simulink model "simulacaoOrientacaoESC"  (R2015a)
settings: Solver=ode4  StartTime=0.0  StopTime=60  FixedStep=0.0001  RelTol=1e-3
values from neighbouring files (symbols this model uses):
  ampSenoide = 15    [simuOrientacaoESC.m]
  freqSenoide = 1.5*2*pi    (= 9.42477796077)    [simuOrientacaoESC.m]
  K = 1    [simuOrientacaoESC.m]
  Kp = 10    [simuOrientacaoESC.m]
undefined symbols (not defined in the file or in its folder): xL0
libraries: simulink_extras x3
settings Model: Creator=Jean  LastModifiedBy=Jean

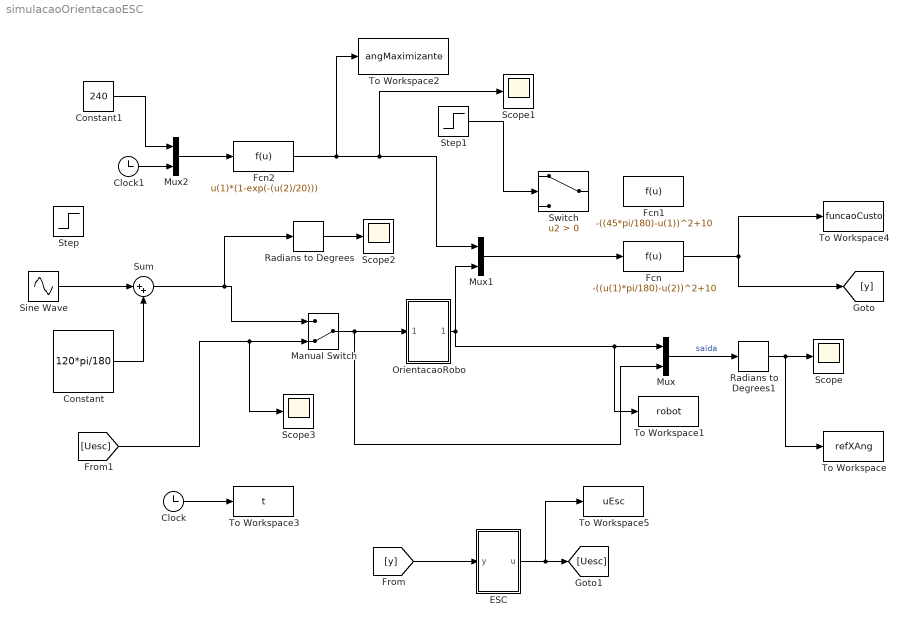
== system simulacaoOrientacaoESC ==
  Clock : Clock
  Clock1 : Clock
  Constant : Constant  Value=120*pi/180
  Constant1 : Constant  Value=240
  ESC : Subsystem
  Fcn : Fcn  Expr=-((u(1)*pi/180)-u(2))^2+10
  Fcn1 : Fcn  Expr=-((45*pi/180)-u(1))^2+10
  Fcn2 : Fcn  Expr=u(1)*(1-exp(-(u(2)/20)))
  Manual Switch : ManualSwitch  CurrentSetting=0
  Mux : Mux  Inputs=2
  Mux1 : Mux  Inputs=2
  Mux2 : Mux  Inputs=2
  "OrientacaoRobo " : Subsystem
  Radians to Degrees : simulink_extras/Transformations/Radians to Degrees
  Radians to Degrees1 : simulink_extras/Transformations/Radians to Degrees
  Scope{,1..3} (4 alike) : Scope
      Scope settings: TimeRange=10  YMin=-80000  YMax=10000
      Scope1 settings: TimeRange=10  YMin=30  YMax=90  SaveName=ScopeData2
      Scope2 settings: TimeRange=10  YMin=-60  YMax=60  SaveName=ScopeData3
      Scope3 settings: TimeRange=10  YMin=20.275  YMax=20.825  SaveName=ScopeData4
  Sine Wave : Sin  Amplitude=60*pi/180  Frequency=180*pi/180  SampleTime=0
  Step : Step  SampleTime=0
  Step1 : Step  Time=10  SampleTime=0
  Sum : Sum  Inputs=|++
  Switch : Switch  Criteria=u2 > Threshold
  To Workspace : ToWorkspace  VariableName=refXAng  SaveFormat=Structure With Time  SampleTime=-1
  To Workspace1 : ToWorkspace  VariableName=robot  SaveFormat=Structure With Time  SampleTime=-1
  To Workspace2 : ToWorkspace  VariableName=angMaximizante  SaveFormat=Structure With Time  SampleTime=-1
  To Workspace3 : ToWorkspace  VariableName=t  SaveFormat=Structure With Time  SampleTime=-1
  To Workspace4 : ToWorkspace  VariableName=funcaoCusto  SaveFormat=Structure With Time  SampleTime=-1
  To Workspace5 : ToWorkspace  VariableName=uEsc  SaveFormat=Structure With Time  SampleTime=-1
  wires:
  Manual Switch/1 -> "OrientacaoRobo "/1(In1), Mux/2
  Mux/1 -> Radians to Degrees1/1  "saida"
  [y] -> ESC/1(y)
  ESC/1(u) -> To Workspace5/1, [Uesc]
  [Uesc] -> Scope3/1, Manual Switch/2
  Radians to Degrees/1 -> Scope2/1
  Sine Wave/1 -> Sum/1
  Sum/1 -> Radians to Degrees/1, Manual Switch/1
  Constant/1 -> Sum/2
  Radians to Degrees1/1 -> To Workspace/1, Scope/1
  "OrientacaoRobo "/1(Out1) -> To Workspace1/1, Mux/1, Mux1/2
  Step1/1 -> Switch/2
  Fcn/1 -> To Workspace4/1, [y]
  Mux1/1 -> Fcn/1
  Clock/1 -> To Workspace3/1
  Fcn2/1 -> To Workspace2/1, Scope1/1, Mux1/1
  Constant1/1 -> Mux2/1
  Clock1/1 -> Mux2/2
  Mux2/1 -> Fcn2/1

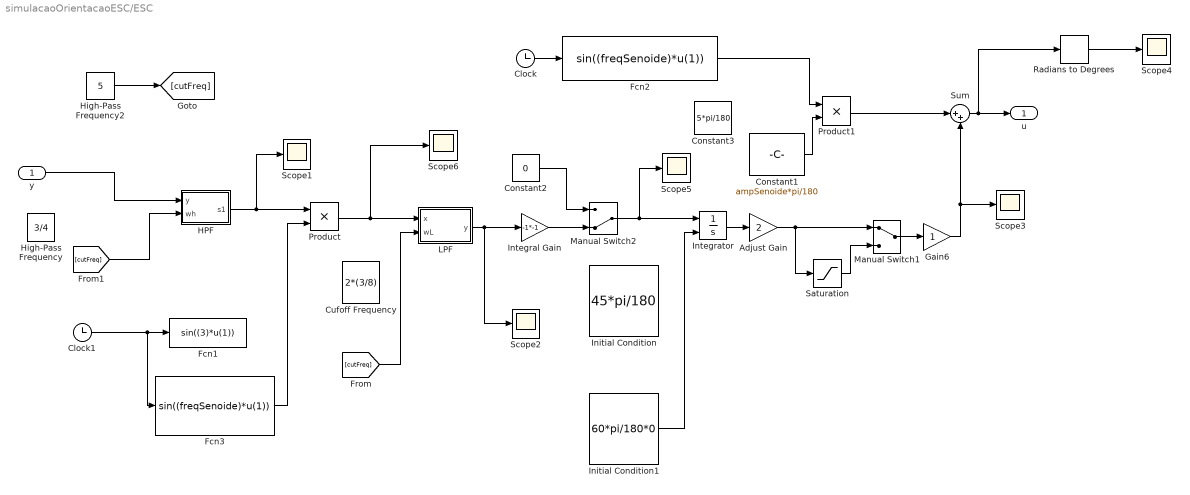
== system simulacaoOrientacaoESC/ESC ==
  y : Inport
  Adjust Gain : Gain  Gain=2
  Clock : Clock
  Clock1 : Clock
  Constant1 : Constant  Value=ampSenoide*pi/180  SampleTime=Inf
  Constant2 : Constant  Value=0
  Constant3 : Constant  Value=5*pi/180  SampleTime=Inf
  Cufoff Frequency : Constant  Value=2*(3/8)  SampleTime=Inf
  Fcn1 : Fcn  Expr=sin((3)*u(1))
  Fcn2 : Fcn  Expr=sin((freqSenoide)*u(1))
  Fcn3 : Fcn  Expr=sin((freqSenoide)*u(1))
  Gain6 : Gain
  HPF : Subsystem
  High-Pass Frequency : Constant  Value=3/4  SampleTime=Inf
  High-Pass Frequency2 : Constant  Value=5  SampleTime=Inf
  Initial Condition : Constant  Value=45*pi/180  SampleTime=Inf
  Initial Condition1 : Constant  Value=60*pi/180*0  SampleTime=Inf
  Integral Gain : Gain  Gain=-1*-1
  Integrator : Integrator  InitialConditionSource=external
  LPF : Subsystem
  Manual Switch1 : ManualSwitch
  Manual Switch2 : ManualSwitch  CurrentSetting=0
  Product : Product
  Product1 : Product
  Radians to Degrees : simulink_extras/Transformations/Radians to Degrees
  Saturation : Saturate  UpperLimit=100  LowerLimit=-100
  Scope{1..6} (6 alike) : Scope
      Scope1 settings: YMin=-0.25  YMax=2.5  SaveName=ScopeData6
      Scope2 settings: YMin=-0.05  YMax=0.08  SaveName=ScopeData8
      Scope3 settings: TimeRange=10  YMin=-900  YMax=0  SaveName=ScopeData9
      Scope4 settings: TimeRange=10  YMin=0.375  YMax=0.65  SaveName=ScopeData10
      Scope5 settings: TimeRange=10  YMin=0.42  YMax=0.56
      Scope6 settings: YMin=-0.2  YMax=0.25  SaveName=ScopeData7
  Sum : Sum  Inputs=|++
  u : Outport
  wires:
  Sum/1 -> u/1, Radians to Degrees/1
  Product1/1 -> Sum/1
  Constant2/1 -> Manual Switch2/1
  Fcn2/1 -> Product1/1
  Integrator/1 -> Adjust Gain/1
  y/1 -> HPF/1(y)
  Gain6/1 -> Sum/2, Scope3/1
  Clock/1 -> Fcn2/1
  Clock1/1 -> Fcn3/1, Fcn1/1
  HPF/1(s1) -> Product/1, Scope1/1
  Adjust Gain/1 -> Saturation/1, Manual Switch1/1
  LPF/1(y) -> Integral Gain/1, Scope2/1
  Integral Gain/1 -> Manual Switch2/2
  Manual Switch1/1 -> Gain6/1
  Manual Switch2/1 -> Scope5/1, Integrator/1
  Saturation/1 -> Manual Switch1/2
  Product/1 -> Scope6/1, LPF/1(x)
  [cutFreq] -> HPF/2(wh)
  Fcn3/1 -> Product/2
  [cutFreq] -> LPF/2(wL)
  Initial Condition1/1 -> Integrator/2
  Constant1/1 -> Product1/2
  Radians to Degrees/1 -> Scope4/1
  High-Pass Frequency2/1 -> [cutFreq]

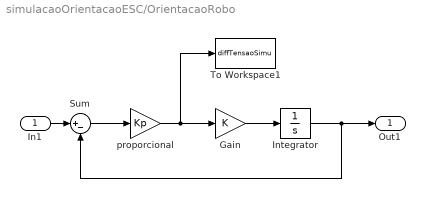
== system simulacaoOrientacaoESC/OrientacaoRobo  ==
  In1 : Inport
  Gain : Gain  Gain=K
  Integrator : Integrator
  Sum : Sum  Inputs=|+-
  To Workspace1 : ToWorkspace  VariableName=diffTensaoSimu  SaveFormat=Structure With Time  SampleTime=-1
  "proporcional " : Gain  Gain=Kp
  Out1 : Outport
  wires:
  Gain/1 -> Integrator/1
  Integrator/1 -> Out1/1, Sum/2
  In1/1 -> Sum/1
  "proporcional "/1 -> To Workspace1/1, Gain/1
  Sum/1 -> "proporcional "/1

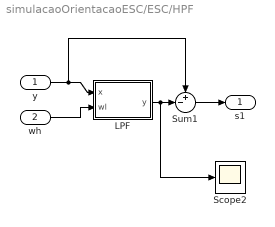
== system simulacaoOrientacaoESC/ESC/HPF ==
  y : Inport
  wh : Inport  Port=2
  LPF : Subsystem
  Scope2 : Scope
      settings: YMin=0.6  YMax=1.125  SaveName=ScopeData5
  Sum1 : Sum  Inputs=+-|
  s1 : Outport
  wires:
  LPF/1(y) -> Sum1/2, Scope2/1
  wh/1 -> LPF/2(wl)
  Sum1/1 -> s1/1
  y/1 -> Sum1/1, LPF/1(x)

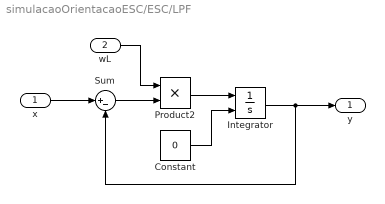
== system simulacaoOrientacaoESC/ESC/LPF ==
  x : Inport
  wL : Inport  Port=2
  Constant : Constant  Value=0
  Integrator : Integrator  InitialConditionSource=external  InitialCondition=xL0
  Product2 : Product
  Sum : Sum  Inputs=|+-
  y : Outport
  wires:
  Constant/1 -> Integrator/2
  x/1 -> Sum/1
  Sum/1 -> Product2/2
  Product2/1 -> Integrator/1
  Integrator/1 -> y/1, Sum/2
  wL/1 -> Product2/1

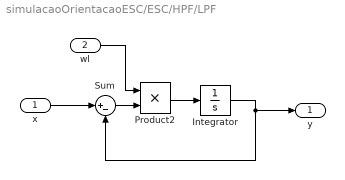
== system simulacaoOrientacaoESC/ESC/HPF/LPF ==
  x : Inport
  wl : Inport  Port=2
  Integrator : Integrator
  Product2 : Product
  Sum : Sum  Inputs=|+-
  y : Outport
  wires:
  wl/1 -> Product2/1
  Integrator/1 -> y/1, Sum/2
  Product2/1 -> Integrator/1
  Sum/1 -> Product2/2
  x/1 -> Sum/1
